simulink model "walkingRobotRL3D"  (R2020b)
settings: Solver=ode23t  StartTime=0.0  StopTime=Tf  RelTol=1e-2  EnableMultiTasking=on
PreLoadFcn:
  | robotParametersRL
undefined symbols (not defined in the file): agent, ankleD_pitch_jointMAX, ankleD_pitch_jointMIN, ankleD_roll_jointMAX, ankleD_roll_jointMIN, ankleI_pitch_jointMAX, ankleI_pitch_jointMIN, ankleI_roll_jointMAX, ankleI_roll_jointMIN, getSampleTime, height_plane, hipD_pitch_jointMAX, hipD_pitch_jointMIN, hipD_roll_jointMAX, hipD_roll_jointMIN, hipI_pitch_jointMAX, hipI_pitch_jointMIN, hipI_roll_jointMAX, hipI_roll_jointMIN, init_angs_L, init_angs_R, init_height, joint_damping, joint_limit_damping, joint_limit_stiffness, joint_stiffness, kneeD_jointMAX, kneeD_jointMIN, kneeI_jointMAX, kneeI_jointMIN, lower_leg_I0, lower_leg_length, lower_leg_mass, lower_leg_x, lower_leg_y, muscle_nominal_length, p10_ankleD_roll, plane_x, plane_y, regulator_type, tau, Tf, torso_height, torso_length, torso_offset_x, torso_offset_z, torso_width, torso_x, torso_y, torso_z, Ts, upper_leg_I0, upper_leg_length, upper_leg_mass, upper_leg_x, upper_leg_y, v10_ankleD_pitch, v10_ankleD_roll, v10_ankleI_pitch, v10_ankleI_roll ... (+41)
libraries: sm_lib x222, simulink x183, nesl_utility x130, walkingRobotUtils x69, rllib x2
(part 11 of 24)

== system walkingRobotRL3D/Walking Robot (Angle based)/Antagonistic PAM Right Leg/ankleD_pitch PAM ==
  V1 : Inport
  V2 : Inport  Port=2
  Constant : Constant
  Constant1 : Constant
  F(x,P) mode (Muscles 1) : MATLAB Function  TreatAsAtomicUnit=on
  F(x,P) mode (Muscles 1)1 : MATLAB Function  TreatAsAtomicUnit=on
  Proportional Regulator (Muscles 1) : MATLAB Function  TreatAsAtomicUnit=on
  Proportional Regulator (Muscles 2) : MATLAB Function  TreatAsAtomicUnit=on
  Spring and damping model : Subsystem
  F1 : Outport
  F2 : Outport  Port=2
  x1 : Outport  Port=3
  x2 : Outport  Port=4
  wires:
  Constant1/1 -> Proportional Regulator (Muscles 2)/2(reg_type)
  F(x,P) mode (Muscles 1)/1(F1) -> F1/1, Spring and damping model/1(F1)
  Proportional Regulator (Muscles 2)/1(p1) -> Spring and damping model/4(P2), F(x,P) mode (Muscles 1)1/1(P2)
  Proportional Regulator (Muscles 1)/1(p1) -> Spring and damping model/3(P1), F(x,P) mode (Muscles 1)/1(P1)
  Spring and damping model/2(x2) -> x2/1, F(x,P) mode (Muscles 1)1/2(x_muscle2)
  Spring and damping model/1(x1) -> x1/1, F(x,P) mode (Muscles 1)/2(x_muscle1)
  F(x,P) mode (Muscles 1)1/1(F2) -> F2/1, Spring and damping model/2(F2)
  Constant/1 -> Proportional Regulator (Muscles 1)/2(reg_type)
  V2/1 -> Proportional Regulator (Muscles 2)/1(V1)
  V1/1 -> Proportional Regulator (Muscles 1)/1(V1)

== system walkingRobotRL3D/Walking Robot (Angle based)/Antagonistic PAM Right Leg/ankleD_roll PAM ==
  V1 : Inport
  V2 : Inport  Port=2
  Constant : Constant
  Constant1 : Constant
  F(x,P) mode (Muscles 1) : MATLAB Function  TreatAsAtomicUnit=on
  F(x,P) mode (Muscles 1)1 : MATLAB Function  TreatAsAtomicUnit=on
  Proportional Regulator (Muscles 1) : MATLAB Function  TreatAsAtomicUnit=on
  Proportional Regulator (Muscles 2) : MATLAB Function  TreatAsAtomicUnit=on
  Spring and damping model : Subsystem
  F1 : Outport
  F2 : Outport  Port=2
  x1 : Outport  Port=3
  x2 : Outport  Port=4
  wires:
  Constant1/1 -> Proportional Regulator (Muscles 2)/2(reg_type)
  F(x,P) mode (Muscles 1)/1(F1) -> F1/1, Spring and damping model/1(F1)
  Proportional Regulator (Muscles 2)/1(p1) -> Spring and damping model/4(P2), F(x,P) mode (Muscles 1)1/1(P2)
  Proportional Regulator (Muscles 1)/1(p1) -> Spring and damping model/3(P1), F(x,P) mode (Muscles 1)/1(P1)
  Spring and damping model/2(x2) -> x2/1, F(x,P) mode (Muscles 1)1/2(x_muscle2)
  Spring and damping model/1(x1) -> x1/1, F(x,P) mode (Muscles 1)/2(x_muscle1)
  F(x,P) mode (Muscles 1)1/1(F2) -> F2/1, Spring and damping model/2(F2)
  Constant/1 -> Proportional Regulator (Muscles 1)/2(reg_type)
  V2/1 -> Proportional Regulator (Muscles 2)/1(V1)
  V1/1 -> Proportional Regulator (Muscles 1)/1(V1)

== system walkingRobotRL3D/Walking Robot (Angle based)/Antagonistic PAM Right Leg/hipD_pitch PAM ==
  V1 : Inport
  V2 : Inport  Port=2
  Constant : Constant
  Constant1 : Constant
  F(x,P) mode (Muscles 1) : MATLAB Function  TreatAsAtomicUnit=on
  F(x,P) mode (Muscles 1)1 : MATLAB Function  TreatAsAtomicUnit=on
  Proportional Regulator (Muscles 1) : MATLAB Function  TreatAsAtomicUnit=on
  Proportional Regulator (Muscles 2) : MATLAB Function  TreatAsAtomicUnit=on
  Spring and damping model : Subsystem
  F1 : Outport
  F2 : Outport  Port=2
  x1 : Outport  Port=3
  x2 : Outport  Port=4
  wires:
  Constant1/1 -> Proportional Regulator (Muscles 2)/2(reg_type)
  F(x,P) mode (Muscles 1)/1(F1) -> F1/1, Spring and damping model/1(F1)
  Proportional Regulator (Muscles 2)/1(p1) -> Spring and damping model/4(P2), F(x,P) mode (Muscles 1)1/1(P2)
  Proportional Regulator (Muscles 1)/1(p1) -> Spring and damping model/3(P1), F(x,P) mode (Muscles 1)/1(P1)
  Spring and damping model/2(x2) -> x2/1, F(x,P) mode (Muscles 1)1/2(x_muscle2)
  Spring and damping model/1(x1) -> x1/1, F(x,P) mode (Muscles 1)/2(x_muscle1)
  F(x,P) mode (Muscles 1)1/1(F2) -> F2/1, Spring and damping model/2(F2)
  Constant/1 -> Proportional Regulator (Muscles 1)/2(reg_type)
  V2/1 -> Proportional Regulator (Muscles 2)/1(V1)
  V1/1 -> Proportional Regulator (Muscles 1)/1(V1)

== system walkingRobotRL3D/Walking Robot (Angle based)/Antagonistic PAM Right Leg/hipD_roll PAM ==
  V1 : Inport
  V2 : Inport  Port=2
  Constant : Constant
  Constant1 : Constant
  F(x,P) mode (Muscles 1) : MATLAB Function  TreatAsAtomicUnit=on
  F(x,P) mode (Muscles 1)1 : MATLAB Function  TreatAsAtomicUnit=on
  Proportional Regulator (Muscles 1) : MATLAB Function  TreatAsAtomicUnit=on
  Proportional Regulator (Muscles 2) : MATLAB Function  TreatAsAtomicUnit=on
  Spring and damping model : Subsystem
  F1 : Outport
  F2 : Outport  Port=2
  x1 : Outport  Port=3
  x2 : Outport  Port=4
  wires:
  Constant1/1 -> Proportional Regulator (Muscles 2)/2(reg_type)
  F(x,P) mode (Muscles 1)/1(F1) -> F1/1, Spring and damping model/1(F1)
  Proportional Regulator (Muscles 2)/1(p1) -> Spring and damping model/4(P2), F(x,P) mode (Muscles 1)1/1(P2)
  Proportional Regulator (Muscles 1)/1(p1) -> Spring and damping model/3(P1), F(x,P) mode (Muscles 1)/1(P1)
  Spring and damping model/2(x2) -> x2/1, F(x,P) mode (Muscles 1)1/2(x_muscle2)
  Spring and damping model/1(x1) -> x1/1, F(x,P) mode (Muscles 1)/2(x_muscle1)
  F(x,P) mode (Muscles 1)1/1(F2) -> F2/1, Spring and damping model/2(F2)
  Constant/1 -> Proportional Regulator (Muscles 1)/2(reg_type)
  V2/1 -> Proportional Regulator (Muscles 2)/1(V1)
  V1/1 -> Proportional Regulator (Muscles 1)/1(V1)

== system walkingRobotRL3D/Walking Robot (Angle based)/Antagonistic PAM Right Leg/kneeD PAM ==
  V1 : Inport
  V2 : Inport  Port=2
  Constant : Constant
  Constant1 : Constant
  F(x,P) mode (Muscles 1) : MATLAB Function  TreatAsAtomicUnit=on
  F(x,P) mode (Muscles 1)1 : MATLAB Function  TreatAsAtomicUnit=on
  Proportional Regulator (Muscles 1) : MATLAB Function  TreatAsAtomicUnit=on
  Proportional Regulator (Muscles 2) : MATLAB Function  TreatAsAtomicUnit=on
  Spring and damping model : Subsystem
  F1 : Outport
  F2 : Outport  Port=2
  x1 : Outport  Port=3
  x2 : Outport  Port=4
  wires:
  Constant1/1 -> Proportional Regulator (Muscles 2)/2(reg_type)
  F(x,P) mode (Muscles 1)/1(F1) -> F1/1, Spring and damping model/1(F1)
  Proportional Regulator (Muscles 2)/1(p1) -> Spring and damping model/4(P2), F(x,P) mode (Muscles 1)1/1(P2)
  Proportional Regulator (Muscles 1)/1(p1) -> Spring and damping model/3(P1), F(x,P) mode (Muscles 1)/1(P1)
  Spring and damping model/2(x2) -> x2/1, F(x,P) mode (Muscles 1)1/2(x_muscle2)
  Spring and damping model/1(x1) -> x1/1, F(x,P) mode (Muscles 1)/2(x_muscle1)
  F(x,P) mode (Muscles 1)1/1(F2) -> F2/1, Spring and damping model/2(F2)
  Constant/1 -> Proportional Regulator (Muscles 1)/2(reg_type)
  V2/1 -> Proportional Regulator (Muscles 2)/1(V1)
  V1/1 -> Proportional Regulator (Muscles 1)/1(V1)

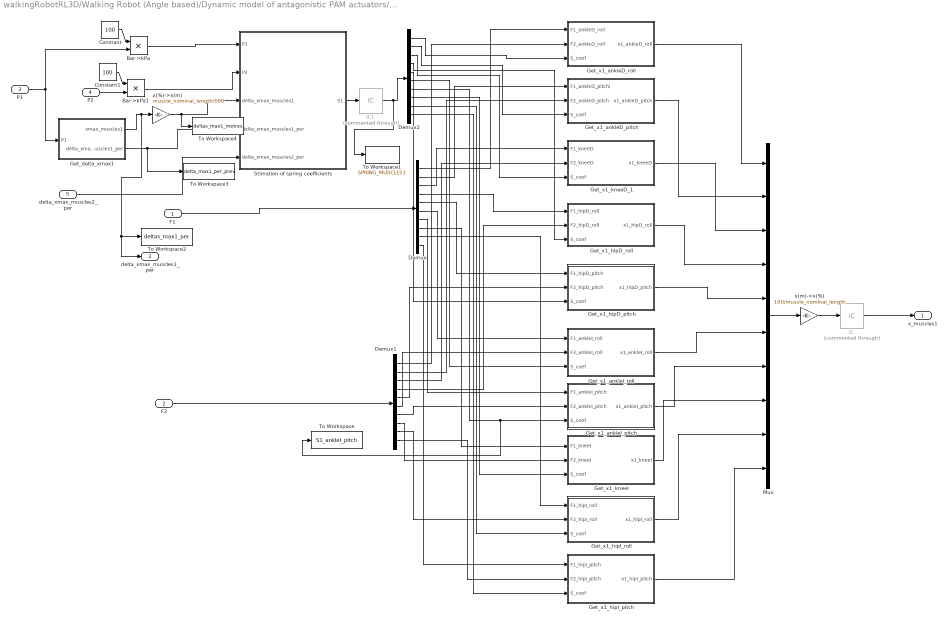
== system walkingRobotRL3D/Walking Robot (Angle based)/Dynamic model of antagonistic PAM actuators/Spring//Damping (Muscles 1) ==
  F1 : Inport
  F2 : Inport  Port=2
  P1 : Inport  Port=3
  P2 : Inport  Port=4
  delta_xmax_muscles2_per : Inport  Port=5
  Bar->kPa : Product
  Bar->kPa1 : Product
  Constant : Constant  Value=100
  Constant1 : Constant  Value=100
  Demux : Demux  Outputs=10
  Demux1 : Demux  Outputs=10
  Demux2 : Demux  Outputs=10
  Get_delta_xmax1 : Subsystem
  Get_x1_ankleD_pitch : Subsystem
  Get_x1_ankleD_roll : Subsystem
  Get_x1_ankleI_pitch : Subsystem
  Get_x1_ankleI_roll : Subsystem
  Get_x1_hipD_pitch : Subsystem
  Get_x1_hipD_roll : Subsystem
  Get_x1_hipI_pitch : Subsystem
  Get_x1_hipI_roll : Subsystem
  Get_x1_kneeD_1 : Subsystem
  Get_x1_kneeI : Subsystem
  IC : InitialCondition  Commented=through  Value=[14.06 0 0 0 0 0]
  IC1 : InitialCondition  Commented=through  Value=[1 1 1 1 1 1 1 1 1 1]'
  Mux : Mux  Inputs=10
  Stimation of spring coefficients : MATLAB Function  TreatAsAtomicUnit=on
  To Workspace : ToWorkspace  VariableName=S1_ankleI_pitch  SaveFormat=Timeseries  SampleTime=-1
  To Workspace1 : ToWorkspace  VariableName=SPRING_MUSCLES1  SaveFormat=Timeseries  SampleTime=-1
  To Workspace2 : ToWorkspace  VariableName=deltas_max1_per  SaveFormat=Timeseries  SampleTime=-1
  To Workspace3 : ToWorkspace  VariableName=delta_max1_per_prev  SaveFormat=Timeseries  SampleTime=-1
  To Workspace4 : ToWorkspace  VariableName=deltas_max1_metres  SaveFormat=Timeseries  SampleTime=-1
  x(%)->x(m) : Gain  Gain=muscle_nominal_length/100
  x(m)->x(%) : Gain  Gain=100/muscle_nominal_length
  x_muscles1 : Outport
  delta_xmax_muscles1_per : Outport  Port=2
  wires:
  Get_delta_xmax1/1(xmax_muscles1) -> To Workspace2/1, delta_xmax_muscles1_per/1, x(%)->x(m)/1
  P1/1 -> Bar->kPa/2, Get_delta_xmax1/1(P1)
  F1/1 -> Demux/1
  x(%)->x(m)/1 -> To Workspace4/1, Stimation of spring coefficients/3(delta_xmax_muscles1)
  Mux/1 -> x(m)->x(%)/1
  x(m)->x(%)/1 -> IC/1
  Stimation of spring coefficients/1(S1) -> IC1/1
  IC/1 -> x_muscles1/1
  Get_x1_ankleD_roll/1(x1_ankleD_roll) -> Mux/1
  Get_x1_ankleD_pitch/1(x1_ankleD_pitch) -> Mux/2
  Get_x1_kneeD_1/1(x1_kneeD) -> Mux/3
  Get_x1_hipD_roll/1(x1_hipD_roll) -> Mux/4
  Get_x1_hipD_pitch/1(x1_hipD_pitch) -> Mux/5
  Get_x1_ankleI_roll/1(x1_ankleI_roll) -> Mux/6
  Get_x1_ankleI_pitch/1(x1_ankleI_pitch) -> Mux/7
  Get_x1_kneeI/1(x1_kneeI) -> Mux/8
  Get_x1_hipI_roll/1(x1_hipI_roll) -> Mux/9
  Get_x1_hipI_pitch/1(x1_hipI_pitch) -> Mux/10
  Demux/1 -> Get_x1_ankleD_roll/1(F1_ankleD_roll)
  Demux/2 -> Get_x1_ankleD_pitch/1(F1_ankleD_pitchl)
  Demux/3 -> Get_x1_kneeD_1/1(F1_kneeD)
  Demux/4 -> Get_x1_hipD_roll/1(F1_hipD_roll)
  Demux/5 -> Get_x1_hipD_pitch/1(F1_hipD_pitch)
  Demux/6 -> Get_x1_ankleI_roll/1(F1_ankleI_roll)
  Demux/7 -> Get_x1_ankleI_pitch/1(F1_ankleI_pitch)
  Demux/8 -> Get_x1_kneeI/1(F1_kneeI)
  Demux/9 -> Get_x1_hipI_roll/1(F1_hipI_roll)
  Demux/10 -> Get_x1_hipI_pitch/1(F1_hipI_pitch)
  Demux1/1 -> Get_x1_ankleD_roll/2(F2_ankleD_roll)
  Demux1/2 -> Get_x1_ankleD_pitch/2(F2_ankleD_pitch)
  Demux1/3 -> Get_x1_kneeD_1/2(F2_kneeD)
  Demux1/4 -> Get_x1_hipD_roll/2(F2_hipD_roll)
  Demux1/5 -> Get_x1_hipD_pitch/2(F2_hipD_pitch)
  Demux1/6 -> Get_x1_ankleI_roll/2(F2_ankleI_roll)
  Demux1/7 -> Get_x1_ankleI_pitch/2(F2_ankleI_pitch)
  Demux1/8 -> Get_x1_kneeI/2(F2_kneeI)
  Demux1/9 -> Get_x1_hipI_roll/2(F2_hipI_roll)
  Demux1/10 -> Get_x1_hipI_pitch/2(F2_hipI_pitch)
  Demux2/1 -> Get_x1_ankleD_roll/3(S_coef)
  Demux2/2 -> Get_x1_ankleD_pitch/3(S_coef)
  Demux2/3 -> Get_x1_kneeD_1/3(S_coef)
  Demux2/4 -> Get_x1_hipD_roll/3(S_coef)
  Demux2/5 -> Get_x1_hipD_pitch/3(S_coef)
  Demux2/6 -> Get_x1_ankleI_roll/3(S_coef)
  Demux2/7 -> To Workspace/1, Get_x1_ankleI_pitch/3(S_coef)
  Demux2/8 -> Get_x1_kneeI/3(S_coef)
  Demux2/9 -> Get_x1_hipI_roll/3(S_coef)
  Demux2/10 -> Get_x1_hipI_pitch/3(S_coef)
  F2/1 -> Demux1/1
  Constant/1 -> Bar->kPa/1
  Bar->kPa/1 -> Stimation of spring coefficients/1(P1)
  Constant1/1 -> Bar->kPa1/1
  P2/1 -> Bar->kPa1/2
  Bar->kPa1/1 -> Stimation of spring coefficients/2(P2)
  delta_xmax_muscles2_per/1 -> Stimation of spring coefficients/5(delta_xmax_muscles2_per)
  Get_delta_xmax1/2(delta_xmax_muscles1_per) -> Stimation of spring coefficients/4(delta_xmax_muscles1_per), To Workspace3/1
  IC1/1 -> To Workspace1/1, Demux2/1

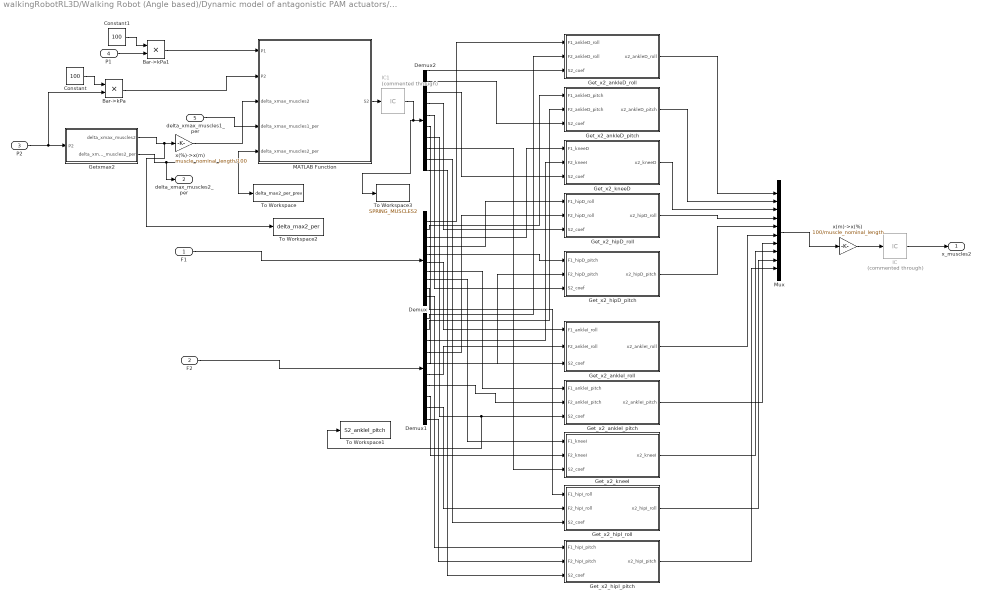
== system walkingRobotRL3D/Walking Robot (Angle based)/Dynamic model of antagonistic PAM actuators/Spring//Damping (Muscles 2) ==
  F1 : Inport
  F2 : Inport  Port=2
  P2 : Inport  Port=3
  P1 : Inport  Port=4
  delta_xmax_muscles1_per : Inport  Port=5
  Bar->kPa : Product
  Bar->kPa1 : Product
  Constant : Constant  Value=100
  Constant1 : Constant  Value=100
  Demux : Demux  Outputs=10
  Demux1 : Demux  Outputs=10
  Demux2 : Demux  Outputs=10
  Get_x2_ankleD_pitch : Subsystem
  Get_x2_ankleD_roll : Subsystem
  Get_x2_ankleI_pitch : Subsystem
  Get_x2_ankleI_roll : Subsystem
  Get_x2_hipD_pitch : Subsystem
  Get_x2_hipD_roll : Subsystem
  Get_x2_hipI_pitch : Subsystem
  Get_x2_hipI_roll : Subsystem
  Get_x2_kneeD : Subsystem
  Get_x2_kneeI : Subsystem
  Getxmax2 : Subsystem
  IC : InitialCondition  Commented=through  Value=[14.06 0 0 0 0 0]
  IC1 : InitialCondition  Commented=through  Value=[1 1 1 1 1 1 1 1 1 1]'
  MATLAB Function : MATLAB Function  TreatAsAtomicUnit=on
  Mux : Mux  Inputs=10
  To Workspace : ToWorkspace  VariableName=delta_max2_per_prev  SaveFormat=Timeseries  SampleTime=-1
  To Workspace1 : ToWorkspace  VariableName=S2_ankleI_pitch  SaveFormat=Timeseries  SampleTime=-1
  To Workspace2 : ToWorkspace  VariableName=delta_max2_per  SaveFormat=Timeseries  SampleTime=-1
  To Workspace3 : ToWorkspace  VariableName=SPRING_MUSCLES2  SaveFormat=Timeseries  SampleTime=-1
  x(%)->x(m) : Gain  Gain=muscle_nominal_length/100
  x(m)->x(%) : Gain  Gain=100/muscle_nominal_length
  x_muscles2 : Outport
  delta_xmax_muscles2_per : Outport  Port=2
  wires:
  F1/1 -> Demux/1
  F2/1 -> Demux1/1
  MATLAB Function/1(S2) -> IC1/1
  P2/1 -> Bar->kPa/2, Getxmax2/1(P2)
  Getxmax2/1(delta_xmax_muscles2) -> To Workspace2/1, x(%)->x(m)/1
  x(%)->x(m)/1 -> MATLAB Function/3(delta_xmax_muscles2)
  Mux/1 -> x(m)->x(%)/1
  x(m)->x(%)/1 -> IC/1
  IC/1 -> x_muscles2/1
  Demux2/1 -> Get_x2_ankleD_roll/3(S2_coef)
  Demux2/2 -> Get_x2_ankleD_pitch/3(S2_coef)
  Demux2/3 -> Get_x2_kneeD/3(S2_coef)
  Demux2/4 -> Get_x2_hipD_roll/3(S2_coef)
  Demux2/5 -> Get_x2_hipD_pitch/3(S2_coef)
  Demux2/6 -> Get_x2_ankleI_roll/3(S2_coef)
  Demux2/7 -> To Workspace1/1, Get_x2_ankleI_pitch/3(S2_coef)
  Demux2/8 -> Get_x2_kneeI/3(S2_coef)
  Demux2/9 -> Get_x2_hipI_roll/3(S2_coef)
  Demux2/10 -> Get_x2_hipI_pitch/3(S2_coef)
  Demux/1 -> Get_x2_ankleD_roll/1(F1_ankleD_roll)
  Demux/2 -> Get_x2_ankleD_pitch/1(F1_ankleD_pitch)
  Demux/3 -> Get_x2_kneeD/1(F1_kneeD)
  Demux/4 -> Get_x2_hipD_roll/1(F1_hipD_roll)
  Demux/5 -> Get_x2_hipD_pitch/1(F1_hipD_pitch)
  Demux/6 -> Get_x2_ankleI_roll/1(F1_ankleI_roll)
  Demux/7 -> Get_x2_ankleI_pitch/1(F1_ankleI_pitch)
  Demux/8 -> Get_x2_kneeI/1(F1_kneeI)
  Demux/9 -> Get_x2_hipI_roll/1(F1_hipI_roll)
  Demux/10 -> Get_x2_hipI_pitch/1(F1_hipI_pitch)
  Demux1/1 -> Get_x2_ankleD_roll/2(F2_ankleD_roll)
  Demux1/2 -> Get_x2_ankleD_pitch/2(F2_ankleD_pitch)
  Demux1/3 -> Get_x2_kneeD/2(F2_kneeI)
  Demux1/4 -> Get_x2_hipD_roll/2(F2_hipD_roll)
  Demux1/5 -> Get_x2_hipD_pitch/2(F2_hipD_pitch)
  Demux1/6 -> Get_x2_ankleI_roll/2(F2_ankleI_roll)
  Demux1/7 -> Get_x2_ankleI_pitch/2(F2_ankleI_pitch)
  Demux1/8 -> Get_x2_kneeI/2(F2_kneeI)
  Demux1/9 -> Get_x2_hipI_roll/2(F2_hipI_roll)
  Demux1/10 -> Get_x2_hipI_pitch/2(F2_hipI_pitch)
  Get_x2_ankleD_roll/1(x2_ankleD_roll) -> Mux/1
  Get_x2_ankleD_pitch/1(x2_ankleD_pitch) -> Mux/2
  Get_x2_kneeD/1(x2_kneeD) -> Mux/3
  Get_x2_hipD_roll/1(x2_hipD_roll) -> Mux/4
  Get_x2_hipD_pitch/1(x2_hipD_pitch) -> Mux/5
  Get_x2_ankleI_roll/1(x2_ankleI_roll) -> Mux/6
  Get_x2_ankleI_pitch/1(x2_ankleI_pitch) -> Mux/7
  Get_x2_kneeI/1(x2_kneeI) -> Mux/8
  Get_x2_hipI_roll/1(x2_hipI_roll) -> Mux/9
  Get_x2_hipI_pitch/1(x2_hipI_pitch) -> Mux/10
  Constant/1 -> Bar->kPa/1
  Bar->kPa/1 -> MATLAB Function/2(P2)
  Constant1/1 -> Bar->kPa1/1
  P1/1 -> Bar->kPa1/2
  Bar->kPa1/1 -> MATLAB Function/1(P1)
  Getxmax2/2(delta_xmax_muscles2_per) -> delta_xmax_muscles2_per/1, To Workspace/1, MATLAB Function/5(delta_xmax_muscles2_per)
  delta_xmax_muscles1_per/1 -> MATLAB Function/4(delta_xmax_muscles1_per)
  IC1/1 -> To Workspace3/1, Demux2/1

== system walkingRobotRL3D/Walking Robot (Angle based)/Robot Leg L/Ankle Pitch Joint ==
  t : Inport
  Bus Creator : BusCreator  Inputs=3
  PS-Simulink Converter1 : nesl_utility/PS-Simulink Converter  PhysicalDomain=network_engine_domain  SubClassName=ps_output  LeftPortType=input  RightPortType=output  PseudoPeriodic=off  Frequencies=[]  Unit=N*m  AffineConversion=off
  PS-Simulink Converter2 : nesl_utility/PS-Simulink Converter  PhysicalDomain=network_engine_domain  SubClassName=ps_output  LeftPortType=input  RightPortType=output  PseudoPeriodic=off  Frequencies=[]  Unit=rad/s  AffineConversion=off
  Revolute Joint : sm_lib/Joints/Revolute Joint  JointMode=Normal  SenseConstraintForce=off  SenseConstraintForceX=off  SenseConstraintForceY=off  SenseConstraintForceZ=off  SenseConstraintTorque=off  SenseConstraintTorqueX=off  SenseConstraintTorqueY=off  SenseConstraintTorqueZ=off  SenseTotalForce=off  SenseTotalForceX=off  SenseTotalForceY=off  SenseTotalForceZ=off  SenseTotalTorque=off  SenseTotalTorqueX=off  SenseTotalTorqueY=off  SenseTotalTorqueZ=off  CompositeWrenchDir=FollowerOnBase  CompositeWrenchFrame=BaseFrame  EquilibriumPosition=eqAngle  EquilibriumPositionUnits=rad  SpringStiffness=k  SpringStiffnessUnits=N*m/rad  DampingCoefficient=d  DampingCoefficientUnits=N*m/(rad/s)  TorqueActuationMode=ComputedTorque  MotionActuationMode=InputMotion  SensePosition=off  SenseVelocity=on  SenseAcceleration=off  SenseTorqueForce=on  SenseLowerLimitTorqueForce=off  SenseUpperLimitTorqueForce=off  LowerLimitSpecify=on  LowerLimitBound=lowerLimit  LowerLimitBoundUnits=rad  LowerLimitStiffness=jointLimitStiffness  LowerLimitStiffnessUnits=N*m/rad  LowerLimitDamping=jointLimitDamping  LowerLimitDampingUnits=N*m/(rad/s)  LowerLimitTransitionRegionWidth=1  LowerLimitTransitionRegionWidthUnits=deg  UpperLimitSpecify=on  UpperLimitBound=upperLimit  UpperLimitBoundUnits=rad  UpperLimitStiffness=jointLimitStiffness  UpperLimitStiffnessUnits=N*m/rad  UpperLimitDamping=jointLimitDamping  UpperLimitDampingUnits=N*m/(rad/s)  UpperLimitTransitionRegionWidth=1  UpperLimitTransitionRegionWidthUnits=deg  PositionTargetSpecify=on  PositionTargetPriority=High  PositionTargetValue=initAngle  PositionTargetValueUnits=rad  VelocityTargetSpecify=off  VelocityTargetPriority=High  VelocityTargetValue=0  VelocityTargetValueUnits=deg/s
  Simulink-PS Converter : nesl_utility/Simulink-PS Converter  PhysicalDomain=network_engine_domain  SubClassName=ps_input  LeftPortType=input  RightPortType=output  PseudoPeriodic=off  Frequencies=[]  NoiseDistribution=none  NoiseParameters=[]  Unit=rad  AffineConversion=off  FilteringAndDerivatives=filter  SimscapeFilterOrder=2  InputFilterTimeConstant=motion_time_constant  UdotUserProvided=0
  B : PMIOPort  Side=Left
  F : PMIOPort  Port=2  Side=Right
  meas : Outport  VectorParamsAs1DForOutWhenUnconnected=off
  wires:
  PS-Simulink Converter1/1 -> Bus Creator/2  "torque"
  Bus Creator/1 -> meas/1
  t/1 -> Bus Creator/1, Simulink-PS Converter/1  "angle"
  PS-Simulink Converter2/1 -> Bus Creator/3  "speed"
  connections:
  Revolute Joint/LConn1 -- B/RConn1
  Revolute Joint/RConn1 -- F/RConn1
  Simulink-PS Converter/RConn1 -- Revolute Joint/LConn2
  Revolute Joint/RConn2 -- PS-Simulink Converter2/LConn1
  Revolute Joint/RConn3 -- PS-Simulink Converter1/LConn1

== system walkingRobotRL3D/Walking Robot (Angle based)/Robot Leg L/Ankle Roll Joint ==
  t : Inport
  Bus Creator : BusCreator  Inputs=3
  PS-Simulink Converter1 : nesl_utility/PS-Simulink Converter  PhysicalDomain=network_engine_domain  SubClassName=ps_output  LeftPortType=input  RightPortType=output  PseudoPeriodic=off  Frequencies=[]  Unit=N*m  AffineConversion=off
  PS-Simulink Converter2 : nesl_utility/PS-Simulink Converter  PhysicalDomain=network_engine_domain  SubClassName=ps_output  LeftPortType=input  RightPortType=output  PseudoPeriodic=off  Frequencies=[]  Unit=rad/s  AffineConversion=off
  Revolute Joint : sm_lib/Joints/Revolute Joint  JointMode=Normal  SenseConstraintForce=off  SenseConstraintForceX=off  SenseConstraintForceY=off  SenseConstraintForceZ=off  SenseConstraintTorque=off  SenseConstraintTorqueX=off  SenseConstraintTorqueY=off  SenseConstraintTorqueZ=off  SenseTotalForce=off  SenseTotalForceX=off  SenseTotalForceY=off  SenseTotalForceZ=off  SenseTotalTorque=off  SenseTotalTorqueX=off  SenseTotalTorqueY=off  SenseTotalTorqueZ=off  CompositeWrenchDir=FollowerOnBase  CompositeWrenchFrame=BaseFrame  EquilibriumPosition=eqAngle  EquilibriumPositionUnits=rad  SpringStiffness=k  SpringStiffnessUnits=N*m/rad  DampingCoefficient=d  DampingCoefficientUnits=N*m/(rad/s)  TorqueActuationMode=ComputedTorque  MotionActuationMode=InputMotion  SensePosition=off  SenseVelocity=on  SenseAcceleration=off  SenseTorqueForce=on  SenseLowerLimitTorqueForce=off  SenseUpperLimitTorqueForce=off  LowerLimitSpecify=on  LowerLimitBound=lowerLimit  LowerLimitBoundUnits=rad  LowerLimitStiffness=jointLimitStiffness  LowerLimitStiffnessUnits=N*m/rad  LowerLimitDamping=jointLimitDamping  LowerLimitDampingUnits=N*m/(rad/s)  LowerLimitTransitionRegionWidth=1  LowerLimitTransitionRegionWidthUnits=deg  UpperLimitSpecify=on  UpperLimitBound=upperLimit  UpperLimitBoundUnits=rad  UpperLimitStiffness=jointLimitStiffness  UpperLimitStiffnessUnits=N*m/rad  UpperLimitDamping=jointLimitDamping  UpperLimitDampingUnits=N*m/(rad/s)  UpperLimitTransitionRegionWidth=1  UpperLimitTransitionRegionWidthUnits=deg  PositionTargetSpecify=on  PositionTargetPriority=High  PositionTargetValue=initAngle  PositionTargetValueUnits=rad  VelocityTargetSpecify=off  VelocityTargetPriority=High  VelocityTargetValue=0  VelocityTargetValueUnits=deg/s
  Simulink-PS Converter : nesl_utility/Simulink-PS Converter  PhysicalDomain=network_engine_domain  SubClassName=ps_input  LeftPortType=input  RightPortType=output  PseudoPeriodic=off  Frequencies=[]  NoiseDistribution=none  NoiseParameters=[]  Unit=rad  AffineConversion=off  FilteringAndDerivatives=filter  SimscapeFilterOrder=2  InputFilterTimeConstant=motion_time_constant  UdotUserProvided=0
  B : PMIOPort  Side=Left
  F : PMIOPort  Port=2  Side=Right
  meas : Outport  VectorParamsAs1DForOutWhenUnconnected=off
  wires:
  PS-Simulink Converter1/1 -> Bus Creator/2  "torque"
  Bus Creator/1 -> meas/1
  t/1 -> Bus Creator/1, Simulink-PS Converter/1  "angle"
  PS-Simulink Converter2/1 -> Bus Creator/3  "speed"
  connections:
  Revolute Joint/LConn1 -- B/RConn1
  Revolute Joint/RConn1 -- F/RConn1
  Simulink-PS Converter/RConn1 -- Revolute Joint/LConn2
  Revolute Joint/RConn2 -- PS-Simulink Converter2/LConn1
  Revolute Joint/RConn3 -- PS-Simulink Converter1/LConn1

== system walkingRobotRL3D/Walking Robot (Angle based)/Robot Leg L/Hip Pitch Joint ==
  t : Inport
  Bus Creator : BusCreator  Inputs=3
  PS-Simulink Converter1 : nesl_utility/PS-Simulink Converter  PhysicalDomain=network_engine_domain  SubClassName=ps_output  LeftPortType=input  RightPortType=output  PseudoPeriodic=off  Frequencies=[]  Unit=N*m  AffineConversion=off
  PS-Simulink Converter2 : nesl_utility/PS-Simulink Converter  PhysicalDomain=network_engine_domain  SubClassName=ps_output  LeftPortType=input  RightPortType=output  PseudoPeriodic=off  Frequencies=[]  Unit=rad/s  AffineConversion=off
  Revolute Joint : sm_lib/Joints/Revolute Joint  JointMode=Normal  SenseConstraintForce=off  SenseConstraintForceX=off  SenseConstraintForceY=off  SenseConstraintForceZ=off  SenseConstraintTorque=off  SenseConstraintTorqueX=off  SenseConstraintTorqueY=off  SenseConstraintTorqueZ=off  SenseTotalForce=off  SenseTotalForceX=off  SenseTotalForceY=off  SenseTotalForceZ=off  SenseTotalTorque=off  SenseTotalTorqueX=off  SenseTotalTorqueY=off  SenseTotalTorqueZ=off  CompositeWrenchDir=FollowerOnBase  CompositeWrenchFrame=BaseFrame  EquilibriumPosition=eqAngle  EquilibriumPositionUnits=rad  SpringStiffness=k  SpringStiffnessUnits=N*m/rad  DampingCoefficient=d  DampingCoefficientUnits=N*m/(rad/s)  TorqueActuationMode=ComputedTorque  MotionActuationMode=InputMotion  SensePosition=off  SenseVelocity=on  SenseAcceleration=off  SenseTorqueForce=on  SenseLowerLimitTorqueForce=off  SenseUpperLimitTorqueForce=off  LowerLimitSpecify=on  LowerLimitBound=lowerLimit  LowerLimitBoundUnits=rad  LowerLimitStiffness=jointLimitStiffness  LowerLimitStiffnessUnits=N*m/rad  LowerLimitDamping=jointLimitDamping  LowerLimitDampingUnits=N*m/(rad/s)  LowerLimitTransitionRegionWidth=1  LowerLimitTransitionRegionWidthUnits=deg  UpperLimitSpecify=on  UpperLimitBound=upperLimit  UpperLimitBoundUnits=rad  UpperLimitStiffness=jointLimitStiffness  UpperLimitStiffnessUnits=N*m/rad  UpperLimitDamping=jointLimitDamping  UpperLimitDampingUnits=N*m/(rad/s)  UpperLimitTransitionRegionWidth=1  UpperLimitTransitionRegionWidthUnits=deg  PositionTargetSpecify=on  PositionTargetPriority=High  PositionTargetValue=initAngle  PositionTargetValueUnits=rad  VelocityTargetSpecify=off  VelocityTargetPriority=High  VelocityTargetValue=0  VelocityTargetValueUnits=deg/s
  Simulink-PS Converter : nesl_utility/Simulink-PS Converter  PhysicalDomain=network_engine_domain  SubClassName=ps_input  LeftPortType=input  RightPortType=output  PseudoPeriodic=off  Frequencies=[]  NoiseDistribution=none  NoiseParameters=[]  Unit=rad  AffineConversion=off  FilteringAndDerivatives=filter  SimscapeFilterOrder=2  InputFilterTimeConstant=motion_time_constant  UdotUserProvided=0
  B : PMIOPort  Side=Left
  F : PMIOPort  Port=2  Side=Right
  meas : Outport  VectorParamsAs1DForOutWhenUnconnected=off
  wires:
  PS-Simulink Converter1/1 -> Bus Creator/2  "torque"
  Bus Creator/1 -> meas/1
  t/1 -> Bus Creator/1, Simulink-PS Converter/1  "angle"
  PS-Simulink Converter2/1 -> Bus Creator/3  "speed"
  connections:
  Revolute Joint/LConn1 -- B/RConn1
  Revolute Joint/RConn1 -- F/RConn1
  Simulink-PS Converter/RConn1 -- Revolute Joint/LConn2
  Revolute Joint/RConn2 -- PS-Simulink Converter2/LConn1
  Revolute Joint/RConn3 -- PS-Simulink Converter1/LConn1

== system walkingRobotRL3D/Walking Robot (Angle based)/Robot Leg L/Hip Roll Joint ==
  t : Inport
  Bus Creator : BusCreator  Inputs=3
  PS-Simulink Converter1 : nesl_utility/PS-Simulink Converter  PhysicalDomain=network_engine_domain  SubClassName=ps_output  LeftPortType=input  RightPortType=output  PseudoPeriodic=off  Frequencies=[]  Unit=N*m  AffineConversion=off
  PS-Simulink Converter2 : nesl_utility/PS-Simulink Converter  PhysicalDomain=network_engine_domain  SubClassName=ps_output  LeftPortType=input  RightPortType=output  PseudoPeriodic=off  Frequencies=[]  Unit=rad/s  AffineConversion=off
  Revolute Joint : sm_lib/Joints/Revolute Joint  JointMode=Normal  SenseConstraintForce=off  SenseConstraintForceX=off  SenseConstraintForceY=off  SenseConstraintForceZ=off  SenseConstraintTorque=off  SenseConstraintTorqueX=off  SenseConstraintTorqueY=off  SenseConstraintTorqueZ=off  SenseTotalForce=off  SenseTotalForceX=off  SenseTotalForceY=off  SenseTotalForceZ=off  SenseTotalTorque=off  SenseTotalTorqueX=off  SenseTotalTorqueY=off  SenseTotalTorqueZ=off  CompositeWrenchDir=FollowerOnBase  CompositeWrenchFrame=BaseFrame  EquilibriumPosition=eqAngle  EquilibriumPositionUnits=rad  SpringStiffness=k  SpringStiffnessUnits=N*m/rad  DampingCoefficient=d  DampingCoefficientUnits=N*m/(rad/s)  TorqueActuationMode=ComputedTorque  MotionActuationMode=InputMotion  SensePosition=off  SenseVelocity=on  SenseAcceleration=off  SenseTorqueForce=on  SenseLowerLimitTorqueForce=off  SenseUpperLimitTorqueForce=off  LowerLimitSpecify=on  LowerLimitBound=lowerLimit  LowerLimitBoundUnits=rad  LowerLimitStiffness=jointLimitStiffness  LowerLimitStiffnessUnits=N*m/rad  LowerLimitDamping=jointLimitDamping  LowerLimitDampingUnits=N*m/(rad/s)  LowerLimitTransitionRegionWidth=1  LowerLimitTransitionRegionWidthUnits=deg  UpperLimitSpecify=on  UpperLimitBound=upperLimit  UpperLimitBoundUnits=rad  UpperLimitStiffness=jointLimitStiffness  UpperLimitStiffnessUnits=N*m/rad  UpperLimitDamping=jointLimitDamping  UpperLimitDampingUnits=N*m/(rad/s)  UpperLimitTransitionRegionWidth=1  UpperLimitTransitionRegionWidthUnits=deg  PositionTargetSpecify=on  PositionTargetPriority=High  PositionTargetValue=initAngle  PositionTargetValueUnits=rad  VelocityTargetSpecify=off  VelocityTargetPriority=High  VelocityTargetValue=0  VelocityTargetValueUnits=deg/s
  Simulink-PS Converter : nesl_utility/Simulink-PS Converter  PhysicalDomain=network_engine_domain  SubClassName=ps_input  LeftPortType=input  RightPortType=output  PseudoPeriodic=off  Frequencies=[]  NoiseDistribution=none  NoiseParameters=[]  Unit=rad  AffineConversion=off  FilteringAndDerivatives=filter  SimscapeFilterOrder=2  InputFilterTimeConstant=motion_time_constant  UdotUserProvided=0
  B : PMIOPort  Side=Left
  F : PMIOPort  Port=2  Side=Right
  meas : Outport  VectorParamsAs1DForOutWhenUnconnected=off
  wires:
  PS-Simulink Converter1/1 -> Bus Creator/2  "torque"
  Bus Creator/1 -> meas/1
  t/1 -> Bus Creator/1, Simulink-PS Converter/1  "angle"
  PS-Simulink Converter2/1 -> Bus Creator/3  "speed"
  connections:
  Revolute Joint/LConn1 -- B/RConn1
  Revolute Joint/RConn1 -- F/RConn1
  Simulink-PS Converter/RConn1 -- Revolute Joint/LConn2
  Revolute Joint/RConn2 -- PS-Simulink Converter2/LConn1
  Revolute Joint/RConn3 -- PS-Simulink Converter1/LConn1

== system walkingRobotRL3D/Walking Robot (Angle based)/Robot Leg L/Knee Joint ==
  t : Inport
  Bus Creator : BusCreator  Inputs=3
  PS-Simulink Converter1 : nesl_utility/PS-Simulink Converter  PhysicalDomain=network_engine_domain  SubClassName=ps_output  LeftPortType=input  RightPortType=output  PseudoPeriodic=off  Frequencies=[]  Unit=N*m  AffineConversion=off
  PS-Simulink Converter2 : nesl_utility/PS-Simulink Converter  PhysicalDomain=network_engine_domain  SubClassName=ps_output  LeftPortType=input  RightPortType=output  PseudoPeriodic=off  Frequencies=[]  Unit=rad/s  AffineConversion=off
  Revolute Joint : sm_lib/Joints/Revolute Joint  JointMode=Normal  SenseConstraintForce=off  SenseConstraintForceX=off  SenseConstraintForceY=off  SenseConstraintForceZ=off  SenseConstraintTorque=off  SenseConstraintTorqueX=off  SenseConstraintTorqueY=off  SenseConstraintTorqueZ=off  SenseTotalForce=off  SenseTotalForceX=off  SenseTotalForceY=off  SenseTotalForceZ=off  SenseTotalTorque=off  SenseTotalTorqueX=off  SenseTotalTorqueY=off  SenseTotalTorqueZ=off  CompositeWrenchDir=FollowerOnBase  CompositeWrenchFrame=BaseFrame  EquilibriumPosition=eqAngle  EquilibriumPositionUnits=rad  SpringStiffness=k  SpringStiffnessUnits=N*m/rad  DampingCoefficient=d  DampingCoefficientUnits=N*m/(rad/s)  TorqueActuationMode=ComputedTorque  MotionActuationMode=InputMotion  SensePosition=off  SenseVelocity=on  SenseAcceleration=off  SenseTorqueForce=on  SenseLowerLimitTorqueForce=off  SenseUpperLimitTorqueForce=off  LowerLimitSpecify=on  LowerLimitBound=lowerLimit  LowerLimitBoundUnits=rad  LowerLimitStiffness=jointLimitStiffness  LowerLimitStiffnessUnits=N*m/rad  LowerLimitDamping=jointLimitDamping  LowerLimitDampingUnits=N*m/(rad/s)  LowerLimitTransitionRegionWidth=1  LowerLimitTransitionRegionWidthUnits=deg  UpperLimitSpecify=on  UpperLimitBound=upperLimit  UpperLimitBoundUnits=rad  UpperLimitStiffness=jointLimitStiffness  UpperLimitStiffnessUnits=N*m/rad  UpperLimitDamping=jointLimitDamping  UpperLimitDampingUnits=N*m/(rad/s)  UpperLimitTransitionRegionWidth=1  UpperLimitTransitionRegionWidthUnits=deg  PositionTargetSpecify=on  PositionTargetPriority=High  PositionTargetValue=initAngle  PositionTargetValueUnits=rad  VelocityTargetSpecify=off  VelocityTargetPriority=High  VelocityTargetValue=0  VelocityTargetValueUnits=deg/s
  Simulink-PS Converter : nesl_utility/Simulink-PS Converter  PhysicalDomain=network_engine_domain  SubClassName=ps_input  LeftPortType=input  RightPortType=output  PseudoPeriodic=off  Frequencies=[]  NoiseDistribution=none  NoiseParameters=[]  Unit=rad  AffineConversion=off  FilteringAndDerivatives=filter  SimscapeFilterOrder=2  InputFilterTimeConstant=motion_time_constant  UdotUserProvided=0
  B : PMIOPort  Side=Left
  F : PMIOPort  Port=2  Side=Right
  meas : Outport  VectorParamsAs1DForOutWhenUnconnected=off
  wires:
  PS-Simulink Converter1/1 -> Bus Creator/2  "torque"
  Bus Creator/1 -> meas/1
  t/1 -> Bus Creator/1, Simulink-PS Converter/1  "angle"
  PS-Simulink Converter2/1 -> Bus Creator/3  "speed"
  connections:
  Revolute Joint/LConn1 -- B/RConn1
  Revolute Joint/RConn1 -- F/RConn1
  Simulink-PS Converter/RConn1 -- Revolute Joint/LConn2
  Revolute Joint/RConn2 -- PS-Simulink Converter2/LConn1
  Revolute Joint/RConn3 -- PS-Simulink Converter1/LConn1

== system walkingRobotRL3D/Walking Robot (Angle based)/Robot Leg R/Ankle Pitch Joint ==
  t : Inport
  Bus Creator : BusCreator  Inputs=3
  PS-Simulink Converter1 : nesl_utility/PS-Simulink Converter  PhysicalDomain=network_engine_domain  SubClassName=ps_output  LeftPortType=input  RightPortType=output  PseudoPeriodic=off  Frequencies=[]  Unit=N*m  AffineConversion=off
  PS-Simulink Converter2 : nesl_utility/PS-Simulink Converter  PhysicalDomain=network_engine_domain  SubClassName=ps_output  LeftPortType=input  RightPortType=output  PseudoPeriodic=off  Frequencies=[]  Unit=rad/s  AffineConversion=off
  Revolute Joint : sm_lib/Joints/Revolute Joint  JointMode=Normal  SenseConstraintForce=off  SenseConstraintForceX=off  SenseConstraintForceY=off  SenseConstraintForceZ=off  SenseConstraintTorque=off  SenseConstraintTorqueX=off  SenseConstraintTorqueY=off  SenseConstraintTorqueZ=off  SenseTotalForce=off  SenseTotalForceX=off  SenseTotalForceY=off  SenseTotalForceZ=off  SenseTotalTorque=off  SenseTotalTorqueX=off  SenseTotalTorqueY=off  SenseTotalTorqueZ=off  CompositeWrenchDir=FollowerOnBase  CompositeWrenchFrame=BaseFrame  EquilibriumPosition=eqAngle  EquilibriumPositionUnits=rad  SpringStiffness=k  SpringStiffnessUnits=N*m/rad  DampingCoefficient=d  DampingCoefficientUnits=N*m/(rad/s)  TorqueActuationMode=ComputedTorque  MotionActuationMode=InputMotion  SensePosition=off  SenseVelocity=on  SenseAcceleration=off  SenseTorqueForce=on  SenseLowerLimitTorqueForce=off  SenseUpperLimitTorqueForce=off  LowerLimitSpecify=on  LowerLimitBound=lowerLimit  LowerLimitBoundUnits=rad  LowerLimitStiffness=jointLimitStiffness  LowerLimitStiffnessUnits=N*m/rad  LowerLimitDamping=jointLimitDamping  LowerLimitDampingUnits=N*m/(rad/s)  LowerLimitTransitionRegionWidth=1  LowerLimitTransitionRegionWidthUnits=deg  UpperLimitSpecify=on  UpperLimitBound=upperLimit  UpperLimitBoundUnits=rad  UpperLimitStiffness=jointLimitStiffness  UpperLimitStiffnessUnits=N*m/rad  UpperLimitDamping=jointLimitDamping  UpperLimitDampingUnits=N*m/(rad/s)  UpperLimitTransitionRegionWidth=1  UpperLimitTransitionRegionWidthUnits=deg  PositionTargetSpecify=on  PositionTargetPriority=High  PositionTargetValue=initAngle  PositionTargetValueUnits=rad  VelocityTargetSpecify=off  VelocityTargetPriority=High  VelocityTargetValue=0  VelocityTargetValueUnits=deg/s
  Simulink-PS Converter : nesl_utility/Simulink-PS Converter  PhysicalDomain=network_engine_domain  SubClassName=ps_input  LeftPortType=input  RightPortType=output  PseudoPeriodic=off  Frequencies=[]  NoiseDistribution=none  NoiseParameters=[]  Unit=rad  AffineConversion=off  FilteringAndDerivatives=filter  SimscapeFilterOrder=2  InputFilterTimeConstant=motion_time_constant  UdotUserProvided=0
  B : PMIOPort  Side=Left
  F : PMIOPort  Port=2  Side=Right
  meas : Outport  VectorParamsAs1DForOutWhenUnconnected=off
  wires:
  PS-Simulink Converter1/1 -> Bus Creator/2  "torque"
  Bus Creator/1 -> meas/1
  t/1 -> Bus Creator/1, Simulink-PS Converter/1  "angle"
  PS-Simulink Converter2/1 -> Bus Creator/3  "speed"
  connections:
  Revolute Joint/LConn1 -- B/RConn1
  Revolute Joint/RConn1 -- F/RConn1
  Simulink-PS Converter/RConn1 -- Revolute Joint/LConn2
  Revolute Joint/RConn3 -- PS-Simulink Converter1/LConn1
  Revolute Joint/RConn2 -- PS-Simulink Converter2/LConn1

== system walkingRobotRL3D/Walking Robot (Angle based)/Robot Leg R/Ankle Roll Joint ==
  t : Inport
  Bus Creator : BusCreator  Inputs=3
  PS-Simulink Converter1 : nesl_utility/PS-Simulink Converter  PhysicalDomain=network_engine_domain  SubClassName=ps_output  LeftPortType=input  RightPortType=output  PseudoPeriodic=off  Frequencies=[]  Unit=N*m  AffineConversion=off
  PS-Simulink Converter2 : nesl_utility/PS-Simulink Converter  PhysicalDomain=network_engine_domain  SubClassName=ps_output  LeftPortType=input  RightPortType=output  PseudoPeriodic=off  Frequencies=[]  Unit=rad/s  AffineConversion=off
  Revolute Joint : sm_lib/Joints/Revolute Joint  JointMode=Normal  SenseConstraintForce=off  SenseConstraintForceX=off  SenseConstraintForceY=off  SenseConstraintForceZ=off  SenseConstraintTorque=off  SenseConstraintTorqueX=off  SenseConstraintTorqueY=off  SenseConstraintTorqueZ=off  SenseTotalForce=off  SenseTotalForceX=off  SenseTotalForceY=off  SenseTotalForceZ=off  SenseTotalTorque=off  SenseTotalTorqueX=off  SenseTotalTorqueY=off  SenseTotalTorqueZ=off  CompositeWrenchDir=FollowerOnBase  CompositeWrenchFrame=BaseFrame  EquilibriumPosition=eqAngle  EquilibriumPositionUnits=rad  SpringStiffness=k  SpringStiffnessUnits=N*m/rad  DampingCoefficient=d  DampingCoefficientUnits=N*m/(rad/s)  TorqueActuationMode=ComputedTorque  MotionActuationMode=InputMotion  SensePosition=off  SenseVelocity=on  SenseAcceleration=off  SenseTorqueForce=on  SenseLowerLimitTorqueForce=off  SenseUpperLimitTorqueForce=off  LowerLimitSpecify=on  LowerLimitBound=ankleD_roll_jointMIN  LowerLimitBoundUnits=rad  LowerLimitStiffness=jointLimitStiffness  LowerLimitStiffnessUnits=N*m/rad  LowerLimitDamping=jointLimitDamping  LowerLimitDampingUnits=N*m/(rad/s)  LowerLimitTransitionRegionWidth=1  LowerLimitTransitionRegionWidthUnits=deg  UpperLimitSpecify=on  UpperLimitBound=ankleD_roll_jointMAX  UpperLimitBoundUnits=rad  UpperLimitStiffness=jointLimitStiffness  UpperLimitStiffnessUnits=N*m/rad  UpperLimitDamping=jointLimitDamping  UpperLimitDampingUnits=N*m/(rad/s)  UpperLimitTransitionRegionWidth=1  UpperLimitTransitionRegionWidthUnits=deg  PositionTargetSpecify=on  PositionTargetPriority=High  PositionTargetValue=initAngle  PositionTargetValueUnits=rad  VelocityTargetSpecify=off  VelocityTargetPriority=High  VelocityTargetValue=0  VelocityTargetValueUnits=deg/s
  Simulink-PS Converter : nesl_utility/Simulink-PS Converter  PhysicalDomain=network_engine_domain  SubClassName=ps_input  LeftPortType=input  RightPortType=output  PseudoPeriodic=off  Frequencies=[]  NoiseDistribution=none  NoiseParameters=[]  Unit=rad  AffineConversion=off  FilteringAndDerivatives=filter  SimscapeFilterOrder=2  InputFilterTimeConstant=motion_time_constant  UdotUserProvided=0
  B : PMIOPort  Side=Left
  F : PMIOPort  Port=2  Side=Right
  meas : Outport  VectorParamsAs1DForOutWhenUnconnected=off
  wires:
  PS-Simulink Converter1/1 -> Bus Creator/2  "torque"
  Bus Creator/1 -> meas/1
  t/1 -> Bus Creator/1, Simulink-PS Converter/1  "angle"
  PS-Simulink Converter2/1 -> Bus Creator/3  "speed"
  connections:
  Revolute Joint/LConn1 -- B/RConn1
  Revolute Joint/RConn1 -- F/RConn1
  Simulink-PS Converter/RConn1 -- Revolute Joint/LConn2
  Revolute Joint/RConn2 -- PS-Simulink Converter2/LConn1
  Revolute Joint/RConn3 -- PS-Simulink Converter1/LConn1

== system walkingRobotRL3D/Walking Robot (Angle based)/Robot Leg R/Hip Pitch Joint ==
  t : Inport
  Bus Creator : BusCreator  Inputs=3
  PS-Simulink Converter1 : nesl_utility/PS-Simulink Converter  PhysicalDomain=network_engine_domain  SubClassName=ps_output  LeftPortType=input  RightPortType=output  PseudoPeriodic=off  Frequencies=[]  Unit=N*m  AffineConversion=off
  PS-Simulink Converter2 : nesl_utility/PS-Simulink Converter  PhysicalDomain=network_engine_domain  SubClassName=ps_output  LeftPortType=input  RightPortType=output  PseudoPeriodic=off  Frequencies=[]  Unit=rad/s  AffineConversion=off
  Revolute Joint : sm_lib/Joints/Revolute Joint  JointMode=Normal  SenseConstraintForce=off  SenseConstraintForceX=off  SenseConstraintForceY=off  SenseConstraintForceZ=off  SenseConstraintTorque=off  SenseConstraintTorqueX=off  SenseConstraintTorqueY=off  SenseConstraintTorqueZ=off  SenseTotalForce=off  SenseTotalForceX=off  SenseTotalForceY=off  SenseTotalForceZ=off  SenseTotalTorque=off  SenseTotalTorqueX=off  SenseTotalTorqueY=off  SenseTotalTorqueZ=off  CompositeWrenchDir=FollowerOnBase  CompositeWrenchFrame=BaseFrame  EquilibriumPosition=eqAngle  EquilibriumPositionUnits=rad  SpringStiffness=k  SpringStiffnessUnits=N*m/rad  DampingCoefficient=d  DampingCoefficientUnits=N*m/(rad/s)  TorqueActuationMode=ComputedTorque  MotionActuationMode=InputMotion  SensePosition=off  SenseVelocity=on  SenseAcceleration=off  SenseTorqueForce=on  SenseLowerLimitTorqueForce=off  SenseUpperLimitTorqueForce=off  LowerLimitSpecify=on  LowerLimitBound=lowerLimit  LowerLimitBoundUnits=rad  LowerLimitStiffness=jointLimitStiffness  LowerLimitStiffnessUnits=N*m/rad  LowerLimitDamping=jointLimitDamping  LowerLimitDampingUnits=N*m/(rad/s)  LowerLimitTransitionRegionWidth=1  LowerLimitTransitionRegionWidthUnits=deg  UpperLimitSpecify=on  UpperLimitBound=upperLimit  UpperLimitBoundUnits=rad  UpperLimitStiffness=jointLimitStiffness  UpperLimitStiffnessUnits=N*m/rad  UpperLimitDamping=jointLimitDamping  UpperLimitDampingUnits=N*m/(rad/s)  UpperLimitTransitionRegionWidth=1  UpperLimitTransitionRegionWidthUnits=deg  PositionTargetSpecify=on  PositionTargetPriority=High  PositionTargetValue=initAngle  PositionTargetValueUnits=rad  VelocityTargetSpecify=off  VelocityTargetPriority=High  VelocityTargetValue=0  VelocityTargetValueUnits=deg/s
  Simulink-PS Converter : nesl_utility/Simulink-PS Converter  PhysicalDomain=network_engine_domain  SubClassName=ps_input  LeftPortType=input  RightPortType=output  PseudoPeriodic=off  Frequencies=[]  NoiseDistribution=none  NoiseParameters=[]  Unit=rad  AffineConversion=off  FilteringAndDerivatives=filter  SimscapeFilterOrder=2  InputFilterTimeConstant=motion_time_constant  UdotUserProvided=0
  B : PMIOPort  Side=Left
  F : PMIOPort  Port=2  Side=Right
  meas : Outport  VectorParamsAs1DForOutWhenUnconnected=off
  wires:
  PS-Simulink Converter1/1 -> Bus Creator/2  "torque"
  Bus Creator/1 -> meas/1
  t/1 -> Bus Creator/1, Simulink-PS Converter/1  "angle"
  PS-Simulink Converter2/1 -> Bus Creator/3  "speed"
  connections:
  Revolute Joint/LConn1 -- B/RConn1
  Revolute Joint/RConn1 -- F/RConn1
  Simulink-PS Converter/RConn1 -- Revolute Joint/LConn2
  Revolute Joint/RConn3 -- PS-Simulink Converter1/LConn1
  Revolute Joint/RConn2 -- PS-Simulink Converter2/LConn1

== system walkingRobotRL3D/Walking Robot (Angle based)/Robot Leg R/Hip Roll Joint ==
  t : Inport
  Bus Creator : BusCreator  Inputs=3
  PS-Simulink Converter1 : nesl_utility/PS-Simulink Converter  PhysicalDomain=network_engine_domain  SubClassName=ps_output  LeftPortType=input  RightPortType=output  PseudoPeriodic=off  Frequencies=[]  Unit=N*m  AffineConversion=off
  PS-Simulink Converter2 : nesl_utility/PS-Simulink Converter  PhysicalDomain=network_engine_domain  SubClassName=ps_output  LeftPortType=input  RightPortType=output  PseudoPeriodic=off  Frequencies=[]  Unit=rad/s  AffineConversion=off
  Revolute Joint : sm_lib/Joints/Revolute Joint  JointMode=Normal  SenseConstraintForce=off  SenseConstraintForceX=off  SenseConstraintForceY=off  SenseConstraintForceZ=off  SenseConstraintTorque=off  SenseConstraintTorqueX=off  SenseConstraintTorqueY=off  SenseConstraintTorqueZ=off  SenseTotalForce=off  SenseTotalForceX=off  SenseTotalForceY=off  SenseTotalForceZ=off  SenseTotalTorque=off  SenseTotalTorqueX=off  SenseTotalTorqueY=off  SenseTotalTorqueZ=off  CompositeWrenchDir=FollowerOnBase  CompositeWrenchFrame=BaseFrame  EquilibriumPosition=eqAngle  EquilibriumPositionUnits=rad  SpringStiffness=k  SpringStiffnessUnits=N*m/rad  DampingCoefficient=d  DampingCoefficientUnits=N*m/(rad/s)  TorqueActuationMode=ComputedTorque  MotionActuationMode=InputMotion  SensePosition=off  SenseVelocity=on  SenseAcceleration=off  SenseTorqueForce=on  SenseLowerLimitTorqueForce=off  SenseUpperLimitTorqueForce=off  LowerLimitSpecify=on  LowerLimitBound=lowerLimit  LowerLimitBoundUnits=rad  LowerLimitStiffness=jointLimitStiffness  LowerLimitStiffnessUnits=N*m/rad  LowerLimitDamping=jointLimitDamping  LowerLimitDampingUnits=N*m/(rad/s)  LowerLimitTransitionRegionWidth=1  LowerLimitTransitionRegionWidthUnits=deg  UpperLimitSpecify=on  UpperLimitBound=upperLimit  UpperLimitBoundUnits=rad  UpperLimitStiffness=jointLimitStiffness  UpperLimitStiffnessUnits=N*m/rad  UpperLimitDamping=jointLimitDamping  UpperLimitDampingUnits=N*m/(rad/s)  UpperLimitTransitionRegionWidth=1  UpperLimitTransitionRegionWidthUnits=deg  PositionTargetSpecify=on  PositionTargetPriority=High  PositionTargetValue=initAngle  PositionTargetValueUnits=rad  VelocityTargetSpecify=off  VelocityTargetPriority=High  VelocityTargetValue=0  VelocityTargetValueUnits=deg/s
  Simulink-PS Converter : nesl_utility/Simulink-PS Converter  PhysicalDomain=network_engine_domain  SubClassName=ps_input  LeftPortType=input  RightPortType=output  PseudoPeriodic=off  Frequencies=[]  NoiseDistribution=none  NoiseParameters=[]  Unit=rad  AffineConversion=off  FilteringAndDerivatives=filter  SimscapeFilterOrder=2  InputFilterTimeConstant=motion_time_constant  UdotUserProvided=0
  B : PMIOPort  Side=Left
  F : PMIOPort  Port=2  Side=Right
  meas : Outport  VectorParamsAs1DForOutWhenUnconnected=off
  wires:
  PS-Simulink Converter1/1 -> Bus Creator/2  "torque"
  Bus Creator/1 -> meas/1
  t/1 -> Bus Creator/1, Simulink-PS Converter/1  "angle"
  PS-Simulink Converter2/1 -> Bus Creator/3  "speed"
  connections:
  Revolute Joint/LConn1 -- B/RConn1
  Revolute Joint/RConn1 -- F/RConn1
  Simulink-PS Converter/RConn1 -- Revolute Joint/LConn2
  Revolute Joint/RConn2 -- PS-Simulink Converter2/LConn1
  Revolute Joint/RConn3 -- PS-Simulink Converter1/LConn1

== system walkingRobotRL3D/Walking Robot (Angle based)/Robot Leg R/Knee Joint ==
  t : Inport
  Bus Creator : BusCreator  Inputs=3
  PS-Simulink Converter1 : nesl_utility/PS-Simulink Converter  PhysicalDomain=network_engine_domain  SubClassName=ps_output  LeftPortType=input  RightPortType=output  PseudoPeriodic=off  Frequencies=[]  Unit=N*m  AffineConversion=off
  PS-Simulink Converter2 : nesl_utility/PS-Simulink Converter  PhysicalDomain=network_engine_domain  SubClassName=ps_output  LeftPortType=input  RightPortType=output  PseudoPeriodic=off  Frequencies=[]  Unit=rad/s  AffineConversion=off
  Revolute Joint : sm_lib/Joints/Revolute Joint  JointMode=Normal  SenseConstraintForce=off  SenseConstraintForceX=off  SenseConstraintForceY=off  SenseConstraintForceZ=off  SenseConstraintTorque=off  SenseConstraintTorqueX=off  SenseConstraintTorqueY=off  SenseConstraintTorqueZ=off  SenseTotalForce=off  SenseTotalForceX=off  SenseTotalForceY=off  SenseTotalForceZ=off  SenseTotalTorque=off  SenseTotalTorqueX=off  SenseTotalTorqueY=off  SenseTotalTorqueZ=off  CompositeWrenchDir=FollowerOnBase  CompositeWrenchFrame=BaseFrame  EquilibriumPosition=eqAngle  EquilibriumPositionUnits=rad  SpringStiffness=k  SpringStiffnessUnits=N*m/rad  DampingCoefficient=d  DampingCoefficientUnits=N*m/(rad/s)  TorqueActuationMode=ComputedTorque  MotionActuationMode=InputMotion  SensePosition=off  SenseVelocity=on  SenseAcceleration=off  SenseTorqueForce=on  SenseLowerLimitTorqueForce=off  SenseUpperLimitTorqueForce=off  LowerLimitSpecify=on  LowerLimitBound=lowerLimit  LowerLimitBoundUnits=rad  LowerLimitStiffness=jointLimitStiffness  LowerLimitStiffnessUnits=N*m/rad  LowerLimitDamping=jointLimitDamping  LowerLimitDampingUnits=N*m/(rad/s)  LowerLimitTransitionRegionWidth=1  LowerLimitTransitionRegionWidthUnits=deg  UpperLimitSpecify=on  UpperLimitBound=upperLimit  UpperLimitBoundUnits=rad  UpperLimitStiffness=jointLimitStiffness  UpperLimitStiffnessUnits=N*m/rad  UpperLimitDamping=jointLimitDamping  UpperLimitDampingUnits=N*m/(rad/s)  UpperLimitTransitionRegionWidth=1  UpperLimitTransitionRegionWidthUnits=deg  PositionTargetSpecify=on  PositionTargetPriority=High  PositionTargetValue=initAngle  PositionTargetValueUnits=rad  VelocityTargetSpecify=off  VelocityTargetPriority=High  VelocityTargetValue=0  VelocityTargetValueUnits=deg/s
  Simulink-PS Converter : nesl_utility/Simulink-PS Converter  PhysicalDomain=network_engine_domain  SubClassName=ps_input  LeftPortType=input  RightPortType=output  PseudoPeriodic=off  Frequencies=[]  NoiseDistribution=none  NoiseParameters=[]  Unit=rad  AffineConversion=off  FilteringAndDerivatives=filter  SimscapeFilterOrder=2  InputFilterTimeConstant=motion_time_constant  UdotUserProvided=0
  B : PMIOPort  Side=Left
  F : PMIOPort  Port=2  Side=Right
  meas : Outport  VectorParamsAs1DForOutWhenUnconnected=off
  wires:
  PS-Simulink Converter1/1 -> Bus Creator/2  "torque"
  Bus Creator/1 -> meas/1
  t/1 -> Bus Creator/1, Simulink-PS Converter/1  "angle"
  PS-Simulink Converter2/1 -> Bus Creator/3  "speed"
  connections:
  Revolute Joint/LConn1 -- B/RConn1
  Revolute Joint/RConn1 -- F/RConn1
  Simulink-PS Converter/RConn1 -- Revolute Joint/LConn2
  Revolute Joint/RConn2 -- PS-Simulink Converter2/LConn1
  Revolute Joint/RConn3 -- PS-Simulink Converter1/LConn1
